simulink model "ring_mod_link"  (R2016b)
settings: Solver=ode15s  StartTime=0.0  StopTime=5e-9  FixedStep=200e-15  MaxStep=50e-15  MinStep=1e-15  RelTol=1e-3  EnableMultiTasking=on
undefined symbols (not defined in the file): fbw_rx, fbw_tx, fos, L, P_laser, Rpd, t_drop, t_in, Tb, Va, VBIAS
libraries: SiPhotonics x6, powerlib_meascontrol x2, commrandsrc2 x1
settings Model: Creator=lins08  LastModifiedBy=lins08
settings SolverCC: InitialStep=50e-15
settings DataIOCC: LimitDataPoints=on  SaveFormat=Array
settings OptimizationCC: LifeSpan=inf
settings DebuggingCC: SFUnexpectedBacktrackingDiag=warning  SFNoUnconditionalDefaultTransitionDiag=warning  SFExecutionAtInitializationDiag=none
settings HardwareCC: ProdBitPerPointer=32  ProdBitPerSizeT=32  ProdBitPerPtrDiffT=32  ProdLargestAtomicFloat=None  ProdIntDivRoundTo=Undefined  ProdEndianess=Unspecified  ProdWordSize=32  ProdHWDeviceType=32-bit Generic
settings ModelReferenceCC: PropagateSignalLabelsOutOfModel=off
settings GRTTargetCC: TargetLangStandard=C89/C90 (ANSI)  GeneratePreprocessorConditionals=Disable all
settings ConfigComp: CovMetricSettings=dw  CovHtmlReporting=on  CovSaveCumulativeToWorkspaceVar=on  CovSaveSingleToWorkspaceVar=on  CovExternalEMLEnable=off

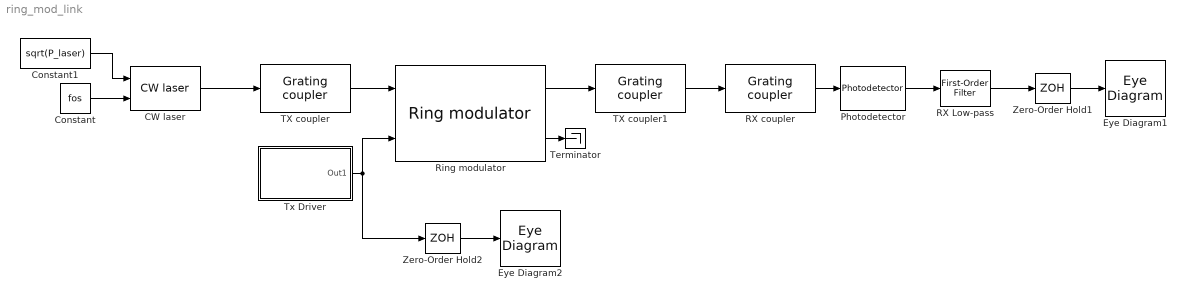
== system ring_mod_link ==
  CW laser : SiPhotonics/CW laser
  Constant : Constant  Value=fos
  Constant1 : Constant  Value=sqrt(P_laser)
  Eye Diagram1 : EyeDiagram
  Eye Diagram2 : EyeDiagram
  Photodetector : SiPhotonics/Photodetector  R=Rpd  fbw=fbw_pd
  RX Low-pass : powerlib_meascontrol/Filters/First-Order Filter  FilterType=Lowpass  Tc=1/(2*pi*fbw_rx)  Ts=0  Initialize=on  Vac_Init=[0, 0, 60]  Vdc_Init=0  PlotResponse=off  FreqRange="[0,  200,  1]"
  RX coupler : SiPhotonics/Grating coupler  trans=Tc
  Ring modulator : SiPhotonics/Ring modulator  L=L  t_in=t_in  k_in=sqrt(1-t_in^2)*1i  t_drop=t_drop  k_drop=sqrt(1-t_drop^2)*1i  fref=fref  n0=n0  ng=ng  n1=n1  a0=a0  a1=a1  Ne=Ne  Nh=Nh  Vbi=Vbi  Lj=Lj  f0=f0  opt=opt  wf=wf
  TX coupler : SiPhotonics/Grating coupler  trans=Tc
  TX coupler1 : SiPhotonics/Grating coupler  trans=Tc
  Terminator : Terminator
  Tx Driver : Subsystem  mask{Va=Va, fbw=fbw_tx, Tb=Tb, Bias=VBIAS}
      mask prompts: Va "Driver output swing"; fbw "Bandwidth"; Tb "Bit width"; Bias "Annode bias"
  Zero-Order Hold1 : ZeroOrderHold  SampleTime=1e-13
  Zero-Order Hold2 : ZeroOrderHold  SampleTime=1e-13
  wires:
  TX coupler/1 -> Ring modulator/1
  Ring modulator/1 -> TX coupler1/1
  RX coupler/1 -> Photodetector/1
  TX coupler1/1 -> RX coupler/1
  CW laser/1 -> TX coupler/1
  Constant/1 -> CW laser/2
  Constant1/1 -> CW laser/1
  Zero-Order Hold1/1 -> Eye Diagram1/1
  Tx Driver/1(Out1) -> Ring modulator/2, Zero-Order Hold2/1
  Zero-Order Hold2/1 -> Eye Diagram2/1
  Ring modulator/2 -> Terminator/1
  Photodetector/1 -> RX Low-pass/1
  RX Low-pass/1 -> Zero-Order Hold1/1

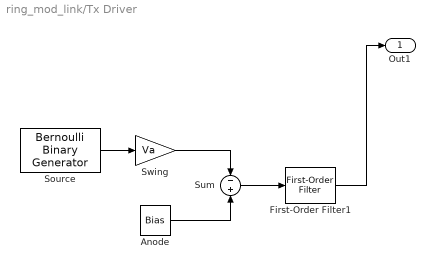
== system ring_mod_link/Tx Driver ==
  Anode : Constant  Value=Bias
  First-Order Filter1 : powerlib_meascontrol/Filters/First-Order Filter  FilterType=Lowpass  Tc=1/(2*pi*fbw)  Ts=0  Initialize=on  Vac_Init=[0, 0, 60]  Vdc_Init=0  PlotResponse=off  FreqRange="[0,  200,  1]"
  Source : commrandsrc2/Bernoulli Binary Generator  P=0.5  seed=61  Ts=Tb  frameBased=off  sampPerFrame=1  orient=off  outDataType=double
  Sum : Sum  Inputs=-+
  Swing : Gain  Gain=Va
  Out1 : Outport
  wires:
  First-Order Filter1/1 -> Out1/1
  Source/1 -> Swing/1
  Swing/1 -> Sum/1
  Sum/1 -> First-Order Filter1/1
  Anode/1 -> Sum/2
